simulink model "fromWorkSpace_TestGen9"  (R2017b)
settings: Solver=FixedStepDiscrete  StartTime=0.0  StopTime=10.0  RelTol=1e-3
model workspace (MAT data in the model file):
  X_timeseries = timeseries
  X_timeseries.Name = 'unnamed'
  X_timeseries.DataInfo = tsdata.datametadata
  X_timeseries.DataInfo.Interpolation = tsdata.interpolation
  X_timeseries.DataInfo.Interpolation.Fhandle : function handle (value not decoded)
  X_timeseries.DataInfo.Interpolation.Name = 'linear'
  X_timeseries.TimeInfo = tsdata.timemetadata
  X_timeseries.TimeInfo.Length = 50
  X_timeseries.TimeInfo.DuplicateTimes = 0
  X_timeseries.TimeInfo.Time_ = [0; 0.2; 0.4; 0.6; 0.8; 1; 1.2; 1.4; 1.6; 1.8; 2; 2.2; 2.4; 2.6; 2.8; 3; 3.2; 3.4; 3.6; 3.8; 4; 4.2; 4.4; 4.6; 4.8; 5; 5.2; 5.4; 5.6; 5.8; 6; 6.2; 6.4; 6.6; 6.8; 7; 7.2; 7.4; 7.6; 7.8; 8; 8.2; 8.4; 8.6; 8.8; 9; 9.2; 9.4; 9.6; 9.8]
  X_timeseries.TimeInfo.Initialized = 1
  X_timeseries.QualityInfo = tsdata.qualmetadata
  X_timeseries.Data_ = [1 1 1 1 1 1 1 1 1 1 1 1 ... (1200 elements, 2x3x4x50)]
undefined symbols (not defined in the file): Block_TestLib, enable
settings Model: Creator=ktrinh  LastModifiedBy=ktrinh
settings DebuggingCC: ParameterOverflowMsg=none

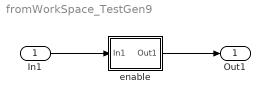
== system fromWorkSpace_TestGen9 ==
  In1 : Inport
  enable : Subsystem  AncestorBlock=Block_TestLib/enable
  Out1 : Outport
  wires:
  In1/1 -> enable/1(In1)
  enable/1(Out1) -> Out1/1

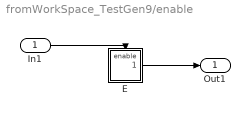
== system fromWorkSpace_TestGen9/enable ==
  In1 : Inport  OutDataTypeStr=boolean
  E : Subsystem  TreatAsAtomicUnit=on
  Out1 : Outport
  wires:
  In1/1 -> E/Enable
  E/1(Out1) -> Out1/1

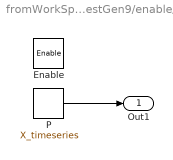
== system fromWorkSpace_TestGen9/enable/E ==
  Enable : EnablePort
  P : FromWorkspace  VariableName=X_timeseries  OutDataTypeStr=boolean  Interpolate=off  OutputAfterFinalValue=Holding final value
  Out1 : Outport
  wires:
  P/1 -> Out1/1
